simulink model "item3_1"  (R2021b)
settings: Solver=VariableStepAuto  StartTime=0.0  StopTime=500  RelTol=1e-3
values from neighbouring files (symbols this model uses):
  dF = 0    [main_proj3.m]
  dTi = 0    [main_proj3.m]
  dTji = 1    [main_proj3.m]
  Fjs = 7.079e-4    (= 0.0007079)    [main_proj3.m]
  Fs = 4.720e-4    (= 0.000472)    [main_proj3.m]
  kp_simc = (1/G011)*(T111/(taoc + L11))    (= 0.000669524614679)    [main_proj3.m]
  Ti_simc = min(T111, 4*(taoc + L11))    [main_proj3.m]
  Tis = 10    [main_proj3.m]
  Tjis = 93.33    [main_proj3.m]
  Tjs = 65.56    [main_proj3.m]
  Ts = 51.67    [main_proj3.m]
libraries: slpidlib x1
settings Model: Creator=henri  LastModifiedBy=luang
settings SolverCC: AlgebraicLoopSolver=TrustRegion
settings DataIOCC: SaveFormat=Array  ReturnWorkspaceOutputs=off  TimeSaveName=tout0  OutputSaveName=yout0
settings DebuggingCC: SFMachineParentedDataDiag=warning
settings SFSimCC: CustomCodeUndefinedFunction=UseInterfaceOnly

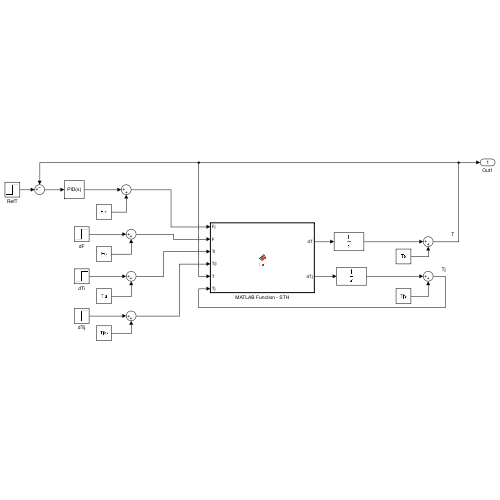
[thumbnail: Simulink's stored preview of the top-level diagram]
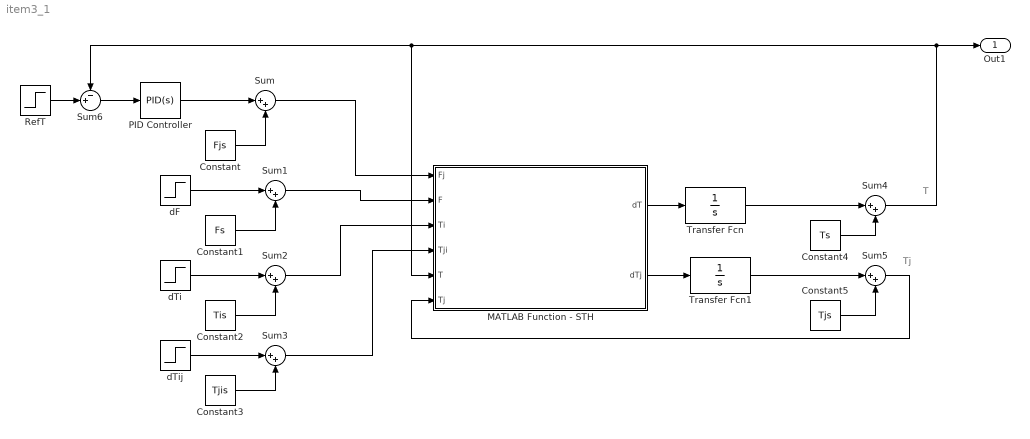
== system item3_1 ==
  note: Tj
  note: T
  Constant : Constant  Value=Fjs
  Constant1 : Constant  Value=Fs
  Constant2 : Constant  Value=Tis
  Constant3 : Constant  Value=Tjis
  Constant4 : Constant  Value=Ts
  Constant5 : Constant  Value=Tjs
  MATLAB Function - STH : MATLAB Function  TreatAsAtomicUnit=on
  PID Controller : slpidlib/PID Controller  Controller=PID  Form=Parallel  TimeDomain=Continuous-time  UseExternalTs=off  SampleTime=-1  IntegratorMethod=Forward Euler  FilterMethod=Forward Euler  ControllerParametersSource=internal  P=kp_simc  I=kp_simc/Ti_simc  D=0  UseFilter=on  N=100  TunerSelectOption=Transfer Function Based (PID Tuner App)  InitialConditionSource=internal  InitialConditionForIntegrator=0  InitialConditionForFilter=0  DifferentiatorICPrevScaledInput=0  ExternalReset=none  TrackingMode=off  Kt=1  LimitOutput=off  SatLimitsSource=internal  UpperSaturationLimit=inf  LowerSaturationLimit=-inf  LinearizeAsGain=on  AntiWindupMode=none  Kb=1  POutMin=[]  POutMax=[]  IOutMin=[]  IOutMax=[]  DOutMin=[]  DOutMax=[]  NOutMin=[]  NOutMax=[]  SumOutMin=[]  SumOutMax=[]  SaturationOutMin=[]  SaturationOutMax=[]  PParamMin=[]  PParamMax=[]  IParamMin=[]  IParamMax=[]  DParamMin=[]  DParamMax=[]  NParamMin=[]  NParamMax=[]  KbParamMin=[]  KbParamMax=[]  KtParamMin=[]  KtParamMax=[]  KbOutMin=[]  KbOutMax=[]  KtOutMin=[]  KtOutMax=[]  IntegratorOutMin=[]  IntegratorOutMax=[]  FilterOutMin=[]  FilterOutMax=[]  SumI1OutMin=[]  SumI1OutMax=[]  SumI2OutMin=[]  SumI2OutMax=[]  SumI3OutMin=[]  SumI3OutMax=[]  SumI4OutMin=[]  SumI4OutMax=[]  SumDOutMin=[]  SumDOutMax=[]  DifferentiatorOutMin=[]  DifferentiatorOutMax=[]  FilterDiffOutCoefMin=[]  FilterDiffOutCoefMax=[]  ReciprocalOutMin=[]  ReciprocalOutMax=[]  SumDenOutMin=[]  SumDenOutMax=[]  SumNumOutMin=[]  SumNumOutMax=[]  DivideOutMin=[]  DivideOutMax=[]  UdiffTsProdOutMin=[]  UdiffTsProdOutMax=[]  NTsProdOutMin=[]  NTsProdOutMax=[]  UintegralTsProdOutMin=[]  UintegralTsProdOutMax=[]  UngainTsProdOutMin=[]  UngainTsProdOutMax=[]  IntegratorContinuousStateAttributes=''  IntegratorStateMustResolveToSignalObject=off  IntegratorRTWStateStorageClass=Auto  FilterContinuousStateAttributes=''  FilterStateMustResolveToSignalObject=off  FilterRTWStateStorageClass=Auto  ParallelPVariant=InternalParameters  IdealPVariant=Disabled  IVariant=InternalParameters  DVariant=InternalParameters  IntegratorVariant=Continuous  SatVariant=Disabled  AWVariant=Passthrough  PCopyVariant=Disabled  TRVariant=Disabled  FdbkBlocksVariant=Forward  IdealPFdbkVariant=Disabled  SatFdbkVariant=Disabled  DerivativeFilterVariant=ContFilter  NVariant=InternalParameters  NCopyVariant=Disabled  FilterICVariant=InternalICsFilter  IntegratorICVariant=InternalICs  ExternalResetVariant=Disabled  TRSumVariant=Passthrough  SumFdbkVariant=Disabled  SumVariant=Sum_PID  TsampFilterVariant=InternalTs  TsampNgainVariant=Passthrough  TsampIntegralVariant=Passthrough  ExternalSaturationOutDataTypeStr=Inherit: Same as second input
  RefT : Step  Time=0  After=Ts  SampleTime=0
  Sum{,1..5} (6 alike) : Sum  Inputs=|++
  Sum6 : Sum  Inputs=-+|
  Transfer Fcn : TransferFcn  Denominator=[1 0]
  Transfer Fcn1 : TransferFcn  Denominator=[1 0]
  dF : Step  Time=0  After=dF  SampleTime=0
  "dTi " : Step  Time=0  After=dTi  SampleTime=0
  dTij : Step  Time=0  After=dTji  SampleTime=0
  Out1 : Outport  VectorParamsAs1DForOutWhenUnconnected=off
  wires:
  MATLAB Function - STH/2(dTj) -> Transfer Fcn1/1
  MATLAB Function - STH/1(dT) -> Transfer Fcn/1
  Transfer Fcn/1 -> Sum4/1
  Constant4/1 -> Sum4/2
  Transfer Fcn1/1 -> Sum5/1
  Constant5/1 -> Sum5/2
  Sum4/1 -> MATLAB Function - STH/5(T), Sum6/1, Out1/1
  Sum5/1 -> MATLAB Function - STH/6(Tj)
  Constant/1 -> Sum/2
  dF/1 -> Sum1/1
  Constant1/1 -> Sum1/2
  Sum/1 -> MATLAB Function - STH/1(Fj)
  Sum1/1 -> MATLAB Function - STH/2(F)
  "dTi "/1 -> Sum2/1
  Constant2/1 -> Sum2/2
  Sum2/1 -> MATLAB Function - STH/3(Ti)
  dTij/1 -> Sum3/1
  Constant3/1 -> Sum3/2
  Sum3/1 -> MATLAB Function - STH/4(Tji)
  PID Controller/1 -> Sum/1
  RefT/1 -> Sum6/2
  Sum6/1 -> PID Controller/1

== matlab function item3_1/MATLAB Function - STH ==
  data: Fj input; dT output; F input; Ti input; Tji input; T input; Tj input; dTj output
function [dT, dTj] = fcn(Fj,F,Ti,Tji,T,Tj)

V = 283.168e-3;
Vj = 28.319e-3;
pcp = 2.165e3;
pcpj = 2.165e3;
UA = 3.065;

dT = ((F/V)*(Ti-T)) + ((UA*(Tj-T))/(V*pcp));
dTj = ((Fj/Vj)*(Tji-Tj)) - ((UA*(Tj-T))/(Vj*pcpj));
